simulink library "lib_EMachine"  (R2017b)
settings: Solver=VariableStepAuto  StartTime=0.0  StopTime=10.0  RelTol=1e-3
undefined symbols (not defined in the file): mot, t_amb, tloop
libraries: simulink x6, lib_Clutch x1
(part 1 of 2)
settings Model: Creator=Di Russo  LastModifiedBy=Vraj M
settings CodeAppCC: StateflowObjectComments=on

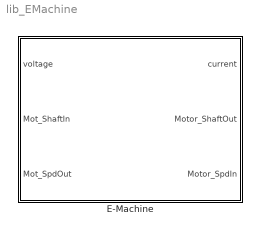
== system lib_EMachine ==
  E-Machine : Subsystem
      mask Display:
      | image('Images/motor.png')
      | color('red');
      | port_label('Input',1,'Volt');
      | port_label('Input',2,'ShaftIn');
      | port_label('Input',3,'SpdOut');
      | port_label('Output',1,'Crr');
      | port_label('Output',2,'ShaftOut');
      | port_label('Output',3,'SpdIn');

== system lib_EMachine/E-Machine ==
  voltage : Inport
  Mot_ShaftIn : Inport  Port=2
  Mot_SpdOut : Inport  Port=3
  Clutch Temporary 1 : Subsystem  Commented=on
  IMG Plant : Subsystem
      mask Display:
      | image('Images\Motor.png')
      | color('red');
      | port_label('Input',2,'Volt');
      | port_label('Input',3,'ShaftIn');
      | port_label('Input',4,'SpdOut');
      | port_label('Output',2,'Crr');
      | port_label('Output',3,'ShaftOut');
      | port_label('Output',4,'SpdIn');
  IMG Plant2 : Subsystem  Commented=on
      mask Display:
      | image('Images/motor.png')
      | color('red');
      | port_label('Input',2,'Volt');
      | port_label('Input',3,'SpdOut');
      | port_label('Input',1,'MCU_cmd');
      | port_label('Input',4,'ShaftIn');
      | port_label('Output',1,'Sensor_Out');
      | port_label('Output',2,'Crr');
      | port_label('Output',3,'MotTrqOut');
      | port_label('Output',4,'MotSpdIn');
  Soft MCU : Subsystem
      mask Display: image('SoftECU.jpg')
  current : Outport
  Motor_ShaftOut : Outport  Port=2
  Motor_SpdIn : Outport  Port=3
  tag scope: MCU_to_HCU=global
  wires:
  IMG Plant/4(SpdIn) -> Motor_SpdIn/1
  Mot_SpdOut/1 -> IMG Plant/4(SpdOut)
  Soft MCU/1(Out) -> [MCU_to_HCU]
  Soft MCU/2(Out1) -> IMG Plant/1("In1 ")  "MCU_to_Actuators"
  [HCU_to_HV_CAN] -> Soft MCU/1(In)
  IMG Plant/1(Out1) -> Soft MCU/2(In1)  "Sensors_to_MCU"
  Mot_ShaftIn/1 -> IMG Plant/3(MotShaftIn)
  IMG Plant/3(MotShaftOut) -> Motor_ShaftOut/1
  voltage/1 -> IMG Plant/2(voltage)
  IMG Plant/2(current) -> current/1

== system lib_EMachine/E-Machine/Clutch Temporary 1 ==
  In1 : Inport
  Constant : Constant  Value=0
  Memory : Memory
  Saturation : Saturate  UpperLimit=inf  LowerLimit=0
  Switch : Switch  Criteria=u2 > Threshold
  Out1 : Outport
  wires:
  Saturation/1 -> Memory/1
  Memory/1 -> Switch/1
  Constant/1 -> Switch/3
  In1/1 -> Saturation/1
  [cltch] -> Switch/2
  Switch/1 -> Out1/1

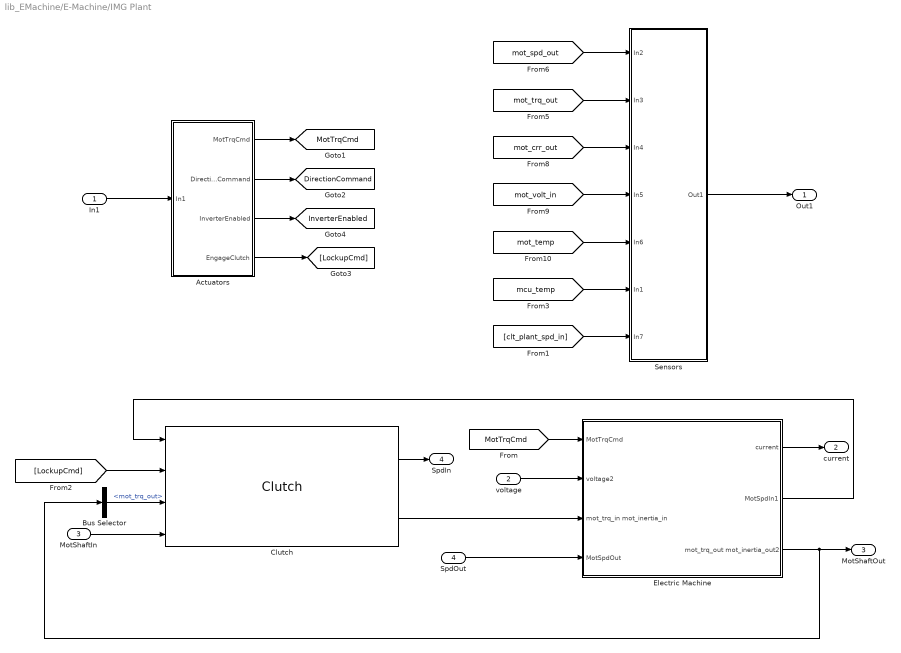
== system lib_EMachine/E-Machine/IMG Plant ==
  "In1 " : Inport
  voltage : Inport  Port=2
  MotShaftIn : Inport  Port=3
  SpdOut : Inport  Port=4
  " Actuators" : Subsystem
  Bus Selector : BusSelector  OutputSignals=mot_trq_out
  Clutch : lib_Clutch/Clutch  SystemSampleTime=-1
  Electric Machine : Subsystem
      mask Display:
      | image('Images\Motor.png')
      | color('red');
      | port_label('Input',1,'MotTrqCmd');
      | port_label('Input',2,'Volt');
      | port_label('Input',3,'ShaftIn');
      | port_label('Input',4,'SpdOut');
      | port_label('Output',1,'Crr')
      | port_label('Output',2,'SpdIn')
  Sensors : Subsystem
  Out1 : Outport
  current : Outport  Port=2
  MotShaftOut : Outport  Port=3
  SpdIn : Outport  Port=4
  tag scope: DirectionCommand=global, InverterEnabled=global, MotTrqCmd=global
  wires:
  Bus Selector/1 -> Clutch/3  "<mot_trq_out>"
  [mot_spd_out] -> Sensors/1(In2)
  [clt_plant_spd_in] -> Sensors/7(In7)
  Clutch/2 -> Electric Machine/3(mot_trq_in mot_inertia_in)
  SpdOut/1 -> Electric Machine/4(MotSpdOut)
  [mcu_temp] -> Sensors/6(In1)
  " Actuators"/3(InverterEnabled) -> [InverterEnabled]
  " Actuators"/2(DirectionCommand) -> [DirectionCommand]
  [LockupCmd] -> Clutch/2
  [mot_temp] -> Sensors/5(In6)
  [mot_crr_out] -> Sensors/3(In4)
  "In1 "/1 -> " Actuators"/1(In1)
  [mot_volt_in] -> Sensors/4(In5)
  " Actuators"/1(MotTrqCmd) -> [MotTrqCmd]
  Sensors/1(Out1) -> Out1/1
  [mot_trq_out] -> Sensors/2(In3)
  Clutch/1 -> SpdIn/1
  Electric Machine/3(mot_trq_out mot_inertia_out2) -> MotShaftOut/1, Bus Selector/1
  MotShaftIn/1 -> Clutch/4
  Electric Machine/2(MotSpdIn1) -> Clutch/1
  Electric Machine/1(current) -> current/1
  [MotTrqCmd] -> Electric Machine/1(MotTrqCmd)
  " Actuators"/4(EngageClutch) -> [LockupCmd]
  voltage/1 -> Electric Machine/2(voltage2)

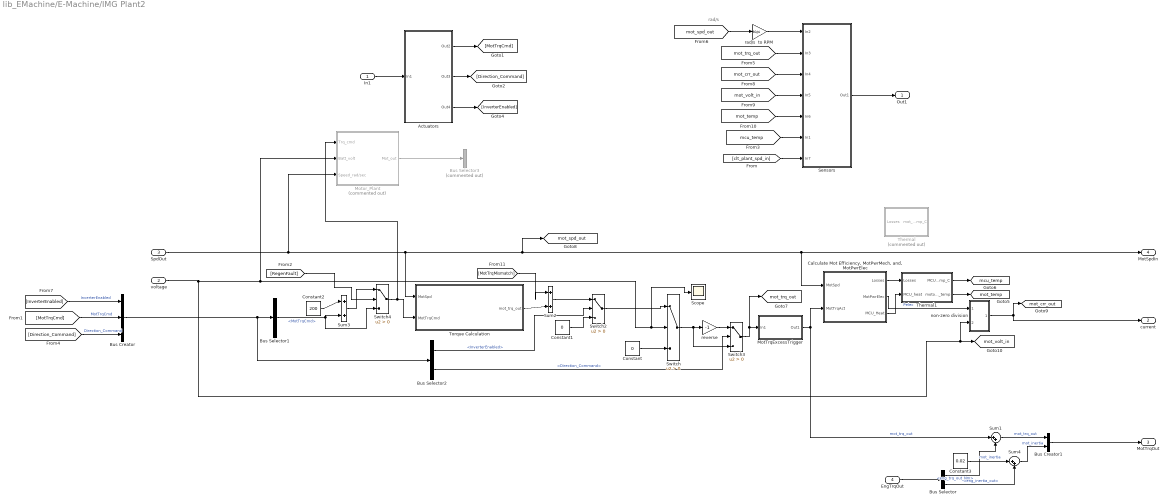
== system lib_EMachine/E-Machine/IMG Plant2 ==
  note: rad/s
  "In1 " : Inport
  voltage : Inport  Port=2
  SpdOut : Inport  Port=3
  EngTrqOut : Inport  Port=4
  " Actuators" : Subsystem
  Bus Creator : BusCreator  Inputs=3
  Bus Creator1 : BusCreator  Inputs=2
  Bus Selector : BusSelector  OutputSignals=eng_trq_out_Nm,eng_inertia_out
  Bus Selector1 : BusSelector  OutputSignals=MotTrqCmd
  Bus Selector2 : BusSelector  OutputSignals=InverterEnabled,Direction_Command
  Bus Selector3 : BusSelector  Commented=on  OutputSignals=Mot_current_A
  "Calculate Mot Efficiency, MotPwrMech, and, MotPwrElec" : Subsystem
  Constant : Constant  Value=0
  Constant1 : Constant  Value=0
  Constant2 : Constant  Value=200
  Constant3 : Constant  Value=0.02
  MotTrqExcessTrigger : Subsystem
  Motor_Plant : Subsystem  Commented=on
  Scope : Scope
  Sensors : Subsystem
  Sum{1..4} (4 alike) : Sum  Inputs=|++
  Switch{,2..4} (4 alike) : Switch  Criteria=u2 > Threshold
  Thermal : Subsystem  Commented=on
  Thermal1 : Subsystem
  Torque Calculation : Subsystem
  non-zero division : Subsystem
      mask Display: disp('divider \n I1/I2')
  rad/s  to RPM : Gain  Gain=30/pi
  reverse : Gain  Gain=-1
  Out1 : Outport
  current : Outport  Port=2
  MotTrqOut : Outport  Port=3
  MotSpdIn : Outport  Port=4
  tag scope: mcu_temp=global, mot_crr_out=global, mot_spd_out=global, mot_temp=global, mot_trq_out=global, mot_volt_in=global
  wires:
  [mot_temp] -> Sensors/5(In6)
  [mot_crr_out] -> Sensors/3(In4)
  "In1 "/1 -> " Actuators"/1(In1)
  [mot_volt_in] -> Sensors/4(In5)
  " Actuators"/1(Out2) -> [MotTrqCmd]
  Sensors/1(Out1) -> Out1/1
  [mot_trq_out] -> Sensors/2(In3)
  SpdOut/1 -> Motor_Plant/3(Speed_rad/sec), Torque Calculation/1(MotSpd), [mot_spd_out], MotSpdIn/1, "Calculate Mot Efficiency, MotPwrMech, and, MotPwrElec"/1(MotSpd)
  non-zero division/1(Out1) -> current/1, [mot_crr_out]
  [mcu_temp] -> Sensors/6(In1)
  [clt_plant_spd_in] -> Sensors/7(In7)
  " Actuators"/2(Out3) -> [Direction_Command]
  " Actuators"/3(Out4) -> [InverterEnabled]
  [Direction_Command] -> Bus Creator/3  "Direction_Command"
  [InverterEnabled] -> Bus Creator/1  "InverterEnabled"
  [MotTrqCmd] -> Bus Creator/2  "MotTrqCmd"
  [mot_spd_out] -> rad/s  to RPM/1
  rad/s  to RPM/1 -> Sensors/1(In2)
  Thermal1/1(MCU_temp_C) -> [mcu_temp]
  Constant2/1 -> Sum3/1
  Switch4/1 -> Motor_Plant/1(Trq_cmd), Torque Calculation/2(MotTrqCmd)
  Sum3/1 -> Switch4/1
  [RegenFault] -> Switch4/2
  Switch3/1 -> [mot_trq_out], MotTrqExcessTrigger/1(In1)
  reverse/1 -> Switch3/1
  Bus Selector2/2 -> Switch3/2  "<Direction_Command>"
  Switch2/1 -> Switch/1
  Constant1/1 -> Switch2/3
  Bus Selector2/1 -> Switch2/2  "<InverterEnabled>"
  Bus Selector1/1 -> Switch4/3, Sum3/2  "<MotTrqCmd>"
  Bus Creator/1 -> Bus Selector2/1, Bus Selector1/1
  Sum2/1 -> Switch2/1
  Torque Calculation/1(mot_trq_out) -> Sum2/2
  [MotTrqMismatch] -> Sum2/1
  Switch/1 -> Switch3/3, reverse/1
  Thermal1/2(motor_temp) -> [mot_temp]
  "Calculate Mot Efficiency, MotPwrMech, and, MotPwrElec"/3(MCU_Heat) -> Thermal1/2(MCU_heat)
  Constant/1 -> Switch/3
  "Calculate Mot Efficiency, MotPwrMech, and, MotPwrElec"/1(Losses) -> Thermal1/1(Losses)
  MotTrqExcessTrigger/1(Out1) -> Sum1/1, "Calculate Mot Efficiency, MotPwrMech, and, MotPwrElec"/2(MotTrqAct)  "mot_trq_out"
  "Calculate Mot Efficiency, MotPwrMech, and, MotPwrElec"/2(MotPwrElec) -> non-zero division/1(In1)  "Pelec"
  voltage/1 -> non-zero division/2(In2), [mot_volt_in], Motor_Plant/2(Batt_volt), Scope/1, Switch/2
  Bus Creator1/1 -> MotTrqOut/1
  Sum4/1 -> Bus Creator1/2  "mot_inertia"
  EngTrqOut/1 -> Bus Selector/1
  Sum1/1 -> Bus Creator1/1  "mot_trq_out"
  Bus Selector/2 -> Sum4/2  "<eng_inertia_out>"
  Constant3/1 -> Sum4/1  "mot_inertia"
  Bus Selector/1 -> Sum1/2  "<eng_trq_out_Nm>"
  Motor_Plant/1(Mot_out) -> Bus Selector3/1

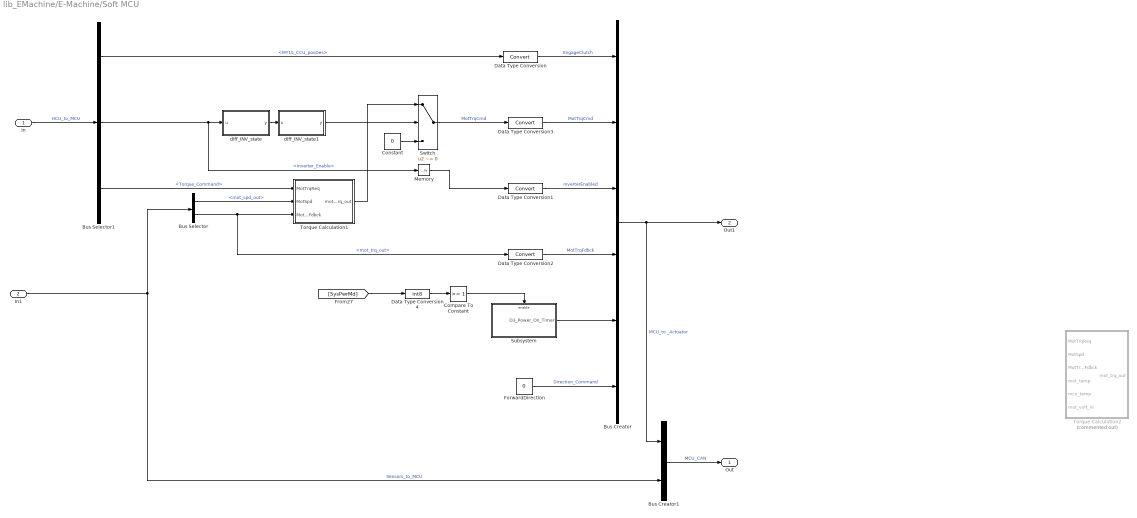
== system lib_EMachine/E-Machine/Soft MCU ==
  In : Inport
  In1 : Inport  Port=2
  Bus Creator : BusCreator  Inputs=6
  Bus Creator1 : BusCreator  Inputs=2
  Bus Selector : BusSelector  OutputSignals=mot_spd_out,mot_trq_out
  Bus Selector1 : BusSelector  OutputSignals=MSG_HYB_115.MY15_CCU_posDes,M192_Command_Message.Inverter_Enable,M192_Command_Message.Torque_Command
  Compare To Constant : simulink/Logic and Bit Operations/Compare To Constant  relop=>=  const=1  OutDataTypeStr=boolean
  Constant : Constant  Value=0
  Data Type Conversion{,1..3} (4 alike) : DataTypeConversion
  Data Type Conversion4 : DataTypeConversion  OutDataTypeStr=int8
  ForwardDirection : Constant  Value=0
  Memory : Memory
  Subsystem : Subsystem
  Switch : Switch  Criteria=u2 ~= 0  Threshold=1
  Torque Calculation1 : Subsystem
  Torque Calculation2 : Subsystem  Commented=on
  diff_INV_state : MATLAB Function  TreatAsAtomicUnit=on
  diff_INV_state1 : MATLAB Function  TreatAsAtomicUnit=on
  Out : Outport
  Out1 : Outport  Port=2
  wires:
  Compare To Constant/1 -> Subsystem/Enable
  Subsystem/1(D3_Power_On_Timer) -> Bus Creator/5
  [SysPwrMd] -> Data Type Conversion4/1
  Data Type Conversion4/1 -> Compare To Constant/1
  Torque Calculation1/1(mot_trq_out) -> Switch/1
  diff_INV_state1/1(y) -> Switch/2
  Bus Selector1/2 -> diff_INV_state/1(u), Memory/1  "<Inverter_Enable>"
  diff_INV_state/1(y) -> diff_INV_state1/1(u)
  ForwardDirection/1 -> Bus Creator/6  "Direction_Command"
  Data Type Conversion3/1 -> Bus Creator/2  "MotTrqCmd"
  Switch/1 -> Data Type Conversion3/1  "MotTrqCmd"
  Memory/1 -> Data Type Conversion1/1
  Data Type Conversion2/1 -> Bus Creator/4  "MotTrqFdbck"
  Bus Selector/2 -> Data Type Conversion2/1, Torque Calculation1/3(MotTrqFdbck)  "<mot_trq_out>"
  Data Type Conversion1/1 -> Bus Creator/3  "InverterEnabled"
  Bus Selector/1 -> Torque Calculation1/2(MotSpd)  "<mot_spd_out>"
  Data Type Conversion/1 -> Bus Creator/1  "EngageClutch"
  Bus Selector1/1 -> Data Type Conversion/1  "<MY15_CCU_posDes>"
  Constant/1 -> Switch/3
  Bus Creator/1 -> Out1/1, Bus Creator1/1  "MCU_to _Actuator"
  Bus Selector1/3 -> Torque Calculation1/1(MotTrqReq)  "<Torque_Command>"
  In/1 -> Bus Selector1/1  "HCU_to_MCU"
  Bus Creator1/1 -> Out/1  "MCU_CAN"
  In1/1 -> Bus Creator1/2, Bus Selector/1  "Sensors_to_MCU"

== system lib_EMachine/E-Machine/IMG Plant/ Actuators ==
  In1 : Inport
  Bus Selector : BusSelector  OutputSignals=MotTrqCmd,Direction_Command,InverterEnabled,EngageClutch
  MotTrqCmd : Outport
  DirectionCommand : Outport  Port=2
  InverterEnabled : Outport  Port=3
  EngageClutch : Outport  Port=4
  wires:
  Bus Selector/3 -> InverterEnabled/1  "<InverterEnabled>"
  Bus Selector/2 -> DirectionCommand/1  "<Direction_Command>"
  Bus Selector/1 -> MotTrqCmd/1  "<MotTrqCmd>"
  In1/1 -> Bus Selector/1
  Bus Selector/4 -> EngageClutch/1  "<EngageClutch>"

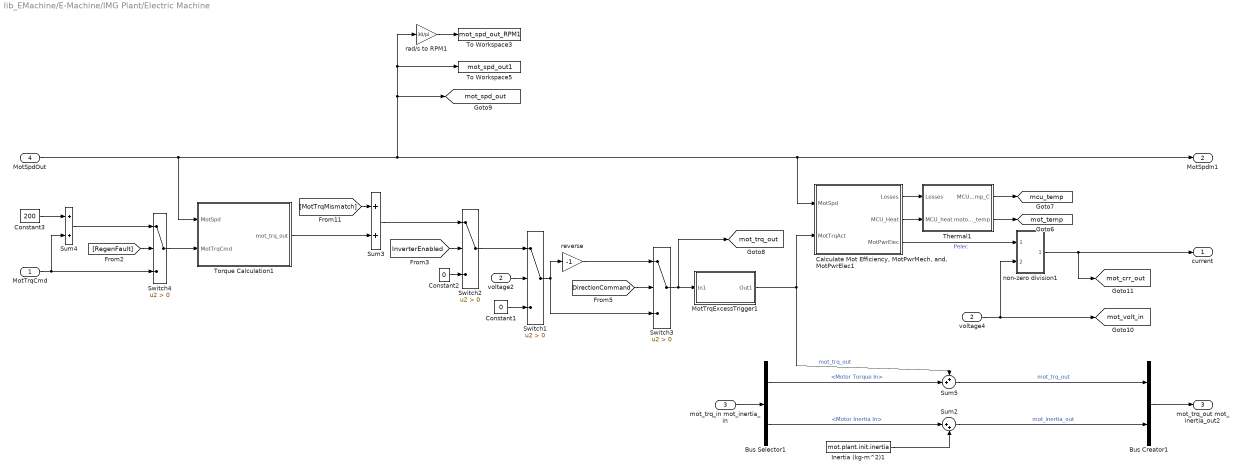
== system lib_EMachine/E-Machine/IMG Plant/Electric Machine ==
  MotTrqCmd : Inport
  voltage2 : Inport  Port=2
  mot_trq_in mot_inertia_in : Inport  Port=3
  MotSpdOut : Inport  Port=4
  Bus Creator1 : BusCreator  Inputs=2
  Bus Selector1 : BusSelector  OutputSignals=Motor Torque In,Motor Inertia In
  "Calculate Mot Efficiency, MotPwrMech, and, MotPwrElec1" : Subsystem
  Constant1 : Constant  Value=0
  Constant2 : Constant  Value=0
  Constant3 : Constant  Value=200
  Inertia (kg-m^2)1 : Constant  Value=mot.plant.init.inertia
  MotTrqExcessTrigger1 : Subsystem
  Sum2 : Sum  Inputs=|++
  Sum3 : Sum
  Sum4 : Sum
  Sum5 : Sum  Inputs=++|
  Switch{1..4} (4 alike) : Switch  Criteria=u2 > Threshold
  Thermal1 : Subsystem
  To Workspace3 : ToWorkspace  VariableName=mot_spd_out_RPM1  SampleTime=-1
      settings: Decimation=WORKSPACE_DECIMATION
  To Workspace5 : ToWorkspace  VariableName=mot_spd_out1  SampleTime=-1
      settings: Decimation=WORKSPACE_DECIMATION
  Torque Calculation1 : Subsystem
  non-zero division1 : Subsystem
      mask Display: disp('divider \n I1/I2')
  rad/s to RPM1 : Gain  Gain=30/pi
  reverse : Gain  Gain=-1
  voltage4 : InportShadow  Port=2
  current : Outport
  MotSpdIn1 : Outport  Port=2
  mot_trq_out mot_inertia_out2 : Outport  Port=3
  tag scope: mcu_temp=global, mot_crr_out=global, mot_spd_out=global, mot_temp=global, mot_trq_out=global, mot_volt_in=global
  wires:
  MotSpdOut/1 -> Torque Calculation1/1(MotSpd), [mot_spd_out], rad/s to RPM1/1, To Workspace5/1, MotSpdIn1/1, "Calculate Mot Efficiency, MotPwrMech, and, MotPwrElec1"/1(MotSpd)
  rad/s to RPM1/1 -> To Workspace3/1
  Bus Selector1/1 -> Sum5/2  "<Motor Torque In>"
  Bus Selector1/2 -> Sum2/1  "<Motor Inertia In>"
  mot_trq_in mot_inertia_in/1 -> Bus Selector1/1
  Bus Creator1/1 -> mot_trq_out mot_inertia_out2/1
  Sum2/1 -> Bus Creator1/2  "mot_inertia_out"
  Inertia (kg-m^2)1/1 -> Sum2/2
  Sum5/1 -> Bus Creator1/1  "mot_trq_out"
  [DirectionCommand] -> Switch3/2
  [InverterEnabled] -> Switch2/2
  [MotTrqMismatch] -> Sum3/1
  voltage4/1 -> [mot_volt_in], non-zero division1/2(In2)
  voltage2/1 -> Switch1/2
  Constant1/1 -> Switch1/3
  Switch1/1 -> Switch3/3, reverse/1
  Constant2/1 -> Switch2/3
  MotTrqCmd/1 -> Switch4/3, Sum4/2
  Sum3/1 -> Switch2/1
  MotTrqExcessTrigger1/1(Out1) -> "Calculate Mot Efficiency, MotPwrMech, and, MotPwrElec1"/2(MotTrqAct), Sum5/1  "mot_trq_out"
  non-zero division1/1(Out1) -> current/1, [mot_crr_out]
  reverse/1 -> Switch3/1
  "Calculate Mot Efficiency, MotPwrMech, and, MotPwrElec1"/3(MotPwrElec) -> non-zero division1/1(In1)  "Pelec"
  Switch4/1 -> Torque Calculation1/2(MotTrqCmd)
  "Calculate Mot Efficiency, MotPwrMech, and, MotPwrElec1"/2(MCU_Heat) -> Thermal1/2(MCU_heat)
  Switch3/1 -> [mot_trq_out], MotTrqExcessTrigger1/1(In1)
  Sum4/1 -> Switch4/1
  "Calculate Mot Efficiency, MotPwrMech, and, MotPwrElec1"/1(Losses) -> Thermal1/1(Losses)
  [RegenFault] -> Switch4/2
  Switch2/1 -> Switch1/1
  Torque Calculation1/1(mot_trq_out) -> Sum3/2
  Constant3/1 -> Sum4/1
  Thermal1/2(motor_temp) -> [mot_temp]
  Thermal1/1(MCU_temp_C) -> [mcu_temp]

== system lib_EMachine/E-Machine/IMG Plant/Sensors ==
  In2 : Inport
  In3 : Inport  Port=2
  In4 : Inport  Port=3
  In5 : Inport  Port=4
  In6 : Inport  Port=5
  In1 : Inport  Port=6
  In7 : Inport  Port=7
  Bus Creator : BusCreator  Inputs=7
  Out1 : Outport
  wires:
  In7/1 -> Bus Creator/7  "clt_plant_spd_in"
  In1/1 -> Bus Creator/6  "mcu_temp"
  In6/1 -> Bus Creator/5  "mot_temp"
  In3/1 -> Bus Creator/2  "mot_trq_out"
  In5/1 -> Bus Creator/4  "mot_volt_in"
  In4/1 -> Bus Creator/3  "mot_crr_out"
  In2/1 -> Bus Creator/1  "mot_spd_out"
  Bus Creator/1 -> Out1/1

== system lib_EMachine/E-Machine/IMG Plant2/ Actuators ==
  In1 : Inport
  Bus Selector : BusSelector  OutputSignals=MotTrqCmd,Direction_Command,InverterEnabled
  Out2 : Outport
  Out3 : Outport  Port=2
  Out4 : Outport  Port=3
  wires:
  Bus Selector/1 -> Out2/1  "<MotTrqCmd>"
  In1/1 -> Bus Selector/1
  Bus Selector/2 -> Out3/1  "<Direction_Command>"
  Bus Selector/3 -> Out4/1  "<InverterEnabled>"

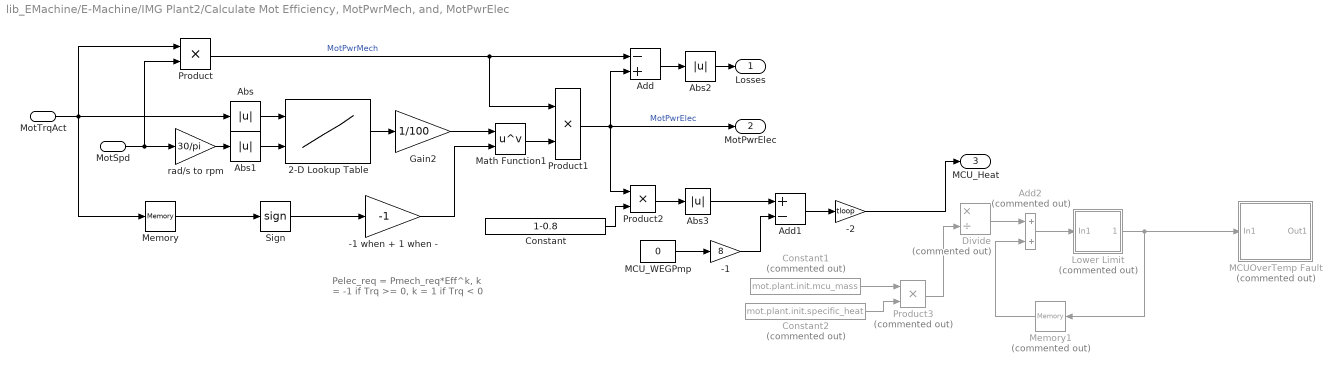
== system lib_EMachine/E-Machine/IMG Plant2/Calculate Mot Efficiency, MotPwrMech, and, MotPwrElec ==
  note: Pelec_req = Pmech_req*Eff^k,
      | k = -1 if Trq >= 0,
      | k = 1 if Trq < 0
  MotSpd : Inport
  MotTrqAct : Inport  Port=2
  -1 : Gain  Gain=8
  "-1 when + 1 when - " : Gain  Gain=-1
  -2 : Gain  Gain=tloop
  2-D Lookup Table : Lookup_n-D  BreakpointsForDimension1=mot.plant.init.eff_trq.idx2_trq  BreakpointsForDimension2=mot.plant.init.eff_trq.idx1_spd  Table=mot.plant.init.eff_trq.map  InternalRulePriority=Speed  RndMeth=Simplest  InputSameDT=on
  Abs{,1..3} (4 alike) : Abs
  Add : Sum  Inputs=-+
  Add1 : Sum  Inputs=+-
  Add2 : Sum  Commented=on
  Constant : Constant  Value=1-0.8
  Constant1 : Constant  Commented=on  Value=mot.plant.init.mcu_mass
  Constant2 : Constant  Commented=on  Value=mot.plant.init.specific_heat
  Divide : Product  Commented=on  Inputs=*/
  Gain2 : Gain  Gain=1/100
  Lower Limit : Subsystem  Commented=on  mask{Lolimit=t_amb+20}
      mask prompts: Lolimit "Lower Limit"
  MCUOverTemp Fault : Subsystem  Commented=on
  MCU_WEGPmp : Constant  Value=0
  Math Function1 : Math  Operator=pow  SaturateOnIntegerOverflow=on
  Memory : Memory
  Memory1 : Memory  Commented=on
  Product : Product
  Product1 : Product
  Product2 : Product
  Product3 : Product  Commented=on
  Sign : Signum
  rad/s to rpm : Gain  Gain=30/pi
  Losses : Outport
  MotPwrElec : Outport  Port=2
  MCU_Heat : Outport  Port=3
  wires:
  rad/s to rpm/1 -> Abs1/1
  Abs1/1 -> 2-D Lookup Table/2
  Sign/1 -> "-1 when + 1 when - "/1
  Abs/1 -> 2-D Lookup Table/1
  Gain2/1 -> Math Function1/1
  2-D Lookup Table/1 -> Gain2/1
  Product1/1 -> Product2/1, Add/2, MotPwrElec/1  "MotPwrElec"
  Product/1 -> Add/1, Product1/1  "MotPwrMech"
  MotTrqAct/1 -> Memory/1, Product/1, Abs/1
  MotSpd/1 -> Product/2, rad/s to rpm/1
  "-1 when + 1 when - "/1 -> Math Function1/2
  Abs2/1 -> Losses/1
  Add/1 -> Abs2/1
  Math Function1/1 -> Product1/2
  Memory/1 -> Sign/1
  Constant/1 -> Product2/2
  Product2/1 -> Abs3/1
  Abs3/1 -> Add1/1
  MCU_WEGPmp/1 -> -1/1
  Add1/1 -> -2/1
  -1/1 -> Add1/2
  -2/1 -> MCU_Heat/1
  Constant1/1 -> Product3/1
  Constant2/1 -> Product3/2
  Product3/1 -> Divide/2
  Divide/1 -> Add2/1
  Memory1/1 -> Add2/2
  Add2/1 -> Lower Limit/1(In1)
  Lower Limit/1(Out1) -> MCUOverTemp Fault/1(In1), Memory1/1

== system lib_EMachine/E-Machine/IMG Plant2/MotTrqExcessTrigger ==
  In1 : Inport
  Bias : Bias  Bias=55
  Bias1 : Bias  Bias=25
  Constant : Constant  Value=0
  Multiport Switch : MultiPortSwitch  DataPortOrder=Zero-based contiguous
  Out1 : Outport
  tag scope: MotTrqExcessTrig=global
  wires:
  Multiport Switch/1 -> Out1/1
  Bias/1 -> Multiport Switch/4
  In1/1 -> Multiport Switch/2, Bias/1, Bias1/1
  Bias1/1 -> Multiport Switch/3
  Constant/1 -> [MotTrqExcessTrig], Multiport Switch/1

== system lib_EMachine/E-Machine/IMG Plant2/Motor_Plant ==
  Trq_cmd : Inport
  Batt_volt : Inport  Port=2
  Speed_rad/sec : Inport  Port=3
  Add : Sum
  Bus Creator : BusCreator  Inputs=5
  Efficiency Calcs : Subsystem
  Memory : Memory
  Random Number : RandomNumber  Mean=0.1  Variance=0.1  SampleTime=0.01
  rad/sec to rpm : Gain  Gain=60/(2*3.14)
  Mot_out : Outport
  wires:
  Add/1 -> Memory/1
  Speed_rad/sec/1 -> rad/sec to rpm/1
  rad/sec to rpm/1 -> Bus Creator/2, Efficiency Calcs/1(Speed_rpm)  "Mot_spd_rpm"
  Random Number/1 -> Add/2
  Memory/1 -> Bus Creator/1, Efficiency Calcs/2(Torq_cmd_Nm)  "Mot_Trq_Nm"
  Bus Creator/1 -> Mot_out/1
  Trq_cmd/1 -> Add/1
  Batt_volt/1 -> Efficiency Calcs/3(Batt_volt)
  Efficiency Calcs/1(Mot_current) -> Bus Creator/3
  Efficiency Calcs/2(Mech_power_W) -> Bus Creator/4
  Efficiency Calcs/3(Elec_power_W) -> Bus Creator/5

== system lib_EMachine/E-Machine/IMG Plant2/Sensors ==
  In2 : Inport
  In3 : Inport  Port=2
  In4 : Inport  Port=3
  In5 : Inport  Port=4
  In6 : Inport  Port=5
  In1 : Inport  Port=6
  In7 : Inport  Port=7
  Bus Creator : BusCreator  Inputs=7
  Out1 : Outport
  wires:
  In6/1 -> Bus Creator/5  "mot_temp"
  In3/1 -> Bus Creator/2  "mot_trq_out"
  In5/1 -> Bus Creator/4  "mot_volt_in"
  In4/1 -> Bus Creator/3  "mot_crr_out"
  In2/1 -> Bus Creator/1  "mot_spd_out"
  Bus Creator/1 -> Out1/1
  In1/1 -> Bus Creator/6  "mcu_temp"
  In7/1 -> Bus Creator/7  "clt_plant_spd_in"

== system lib_EMachine/E-Machine/IMG Plant2/Thermal ==
  Losses : Inport
  Motor Thermal : Subsystem
  mot_temp_C : Outport
  wires:
  Losses/1 -> Motor Thermal/1(In1)  "[W]"
  Motor Thermal/1(Out1) -> mot_temp_C/1

== system lib_EMachine/E-Machine/IMG Plant2/Thermal1 ==
  Losses : Inport
  MCU_heat : Inport  Port=2
  MotInv_loop : Subsystem
  Motor Thermal : Subsystem  Commented=on
  MCU_temp_C : Outport
  motor_temp : Outport  Port=2
  wires:
  MCU_heat/1 -> MotInv_loop/2(In2)
  Losses/1 -> MotInv_loop/1(In1)  "[W]"
  MotInv_loop/1(Out1) -> MCU_temp_C/1
  MotInv_loop/2(Out2) -> motor_temp/1

== system lib_EMachine/E-Machine/IMG Plant2/Torque Calculation ==
  MotSpd : Inport
  MotTrqCmd : Inport  Port=2
  Abs : Abs
  Abs1 : Abs
  MinMax : MinMax  Inputs=2
  Product : Product
  Sign : Signum
  electric machine filter : Subsystem
  "max torque " : Subsystem
  mot_trq_out : Outport
  wires:
  "max torque "/1(max torque) -> Abs1/1
  MotSpd/1 -> "max torque "/2(speed)
  Sign/1 -> Product/1
  MinMax/1 -> Product/2
  Abs/1 -> MinMax/1
  Abs1/1 -> MinMax/2
  electric machine filter/1(filtered) -> mot_trq_out/1
  MotTrqCmd/1 -> "max torque "/1(cmd), Sign/1, Abs/1
  Product/1 -> electric machine filter/1(trq)

== system lib_EMachine/E-Machine/IMG Plant2/non-zero division ==
  note: original idea from Phil Sharer - ANL
      | original formula: u[1]\(u[2]+eps)*(u[2]!=0)
      | changes done by Gerald ZINI (dgey) - ANL (05\02\2001)
  note: (u[2]==0) is true then returns 1, thus (u[2]+(u[2]==0)) is equal to 0+1=1
  note: if u[2] == 0, then output == 0:
  note: (u[2]!=0) is false then returns 0
  note: and finally, the expression is: (u[1] \ 1) * 0 = 0
  note: (u[2]==0) is false then returns 0, thus (u[2]+(u[2]==0)) is equal to u[2]+0=u[2]
  note: if u[2] != 0, then output == u[1]\u[2]:
  note: (u[2]!=0) is true then returns 1
  note: and finally, the expression is: (u[1] \ u[2]) * 1 = u[1] \ u[2]
  In1 : Inport
  In2 : Inport  Port=2
  Fcn : Fcn  Expr=u[1]/(u[2]+(u[2]==0))*(u[2]!=0)
  Mux : Mux  Inputs=2
  Out1 : Outport
  wires:
  Mux/1 -> Fcn/1
  In1/1 -> Mux/1
  Fcn/1 -> Out1/1
  In2/1 -> Mux/2

== system lib_EMachine/E-Machine/Soft MCU/Subsystem ==
  Enable : EnablePort
  MCU_RollingAliveCnt : Subsystem
  D3_Power_On_Timer : Outport
  wires:
  MCU_RollingAliveCnt/1(Out1) -> D3_Power_On_Timer/1  "D3_Power_On_Timer"

== system lib_EMachine/E-Machine/Soft MCU/Torque Calculation1 ==
  MotTrqReq : Inport
  MotSpd : Inport  Port=2
  MotTrqFdbck : Inport  Port=3
  Abs : Abs
  Abs1 : Abs
  MinMax : MinMax  Inputs=2
  Product : Product
  Sign : Signum
  "max torque " : Subsystem
  mot_trq_out : Outport
  wires:
  MotTrqFdbck/1 -> "max torque "/3(torque)
  Abs1/1 -> MinMax/2
  Abs/1 -> MinMax/1
  MinMax/1 -> Product/2
  Sign/1 -> Product/1
  MotTrqReq/1 -> Abs/1, Sign/1, "max torque "/1(Req)
  MotSpd/1 -> "max torque "/2(speed)
  "max torque "/1(max torque) -> Abs1/1
  Product/1 -> mot_trq_out/1

== system lib_EMachine/E-Machine/Soft MCU/Torque Calculation2 ==
  MotTrqReq : Inport
  MotSpd : Inport  Port=2
  MotTrqFdbck : Inport  Port=3
  mot_temp : Inport  Port=4
  mcu_temp : Inport  Port=5
  mot_volt_in : Inport  Port=6
  1-D Lookup Table : Lookup_n-D  NumberOfTableDimensions=1  BreakpointsForDimension1=[0,12600,12700,12800,12900,13000]  Table=[1,1,0.75,0.5,0.25,0]  InternalRulePriority=Speed  RndMeth=Simplest  InputSameDT=on
  1-D Lookup Table1 : Lookup_n-D  NumberOfTableDimensions=1  BreakpointsForDimension1=[0,410,415,420,425,430]  Table=[1,1,0.75,0.5,0.25,0]  InternalRulePriority=Speed  RndMeth=Simplest  InputSameDT=on
  1-D Lookup Table2 : Lookup_n-D  Commented=on  NumberOfTableDimensions=1  BreakpointsForDimension1=[0,90,100]  Table=[1,1,0]  InternalRulePriority=Speed  RndMeth=Simplest  InputSameDT=on
  1-D Lookup Table3 : Lookup_n-D  NumberOfTableDimensions=1  BreakpointsForDimension1=[0,150,170]  Table=[1,1,0]  InternalRulePriority=Speed  RndMeth=Simplest  InputSameDT=on
  Abs : Abs
  Abs1 : Abs
  Constant : Constant
  MinMax : MinMax  Inputs=2
  Product : Product
  Product1 : Product  Inputs=5
  Sign : Signum
  Terminator1 : Terminator
  "max torque " : Subsystem
  rad/s to RPM1 : Gain  Gain=30/pi
  mot_trq_out : Outport
  wires:
  1-D Lookup Table3/1 -> Product1/1
  Constant/1 -> Product1/2
  mcu_temp/1 -> Terminator1/1
  mot_temp/1 -> 1-D Lookup Table3/1
  1-D Lookup Table1/1 -> Product1/3
  mot_volt_in/1 -> 1-D Lookup Table1/1
  1-D Lookup Table/1 -> Product1/4
  Product1/1 -> mot_trq_out/1
  rad/s to RPM1/1 -> 1-D Lookup Table/1
  MotTrqFdbck/1 -> "max torque "/3(torque)
  Abs1/1 -> MinMax/2
  Abs/1 -> MinMax/1
  MinMax/1 -> Product/2
  Sign/1 -> Product/1
  MotTrqReq/1 -> Abs/1, Sign/1, "max torque "/1(Req)
  MotSpd/1 -> "max torque "/2(speed), rad/s to RPM1/1
  "max torque "/1(max torque) -> Abs1/1
  Product/1 -> Product1/5

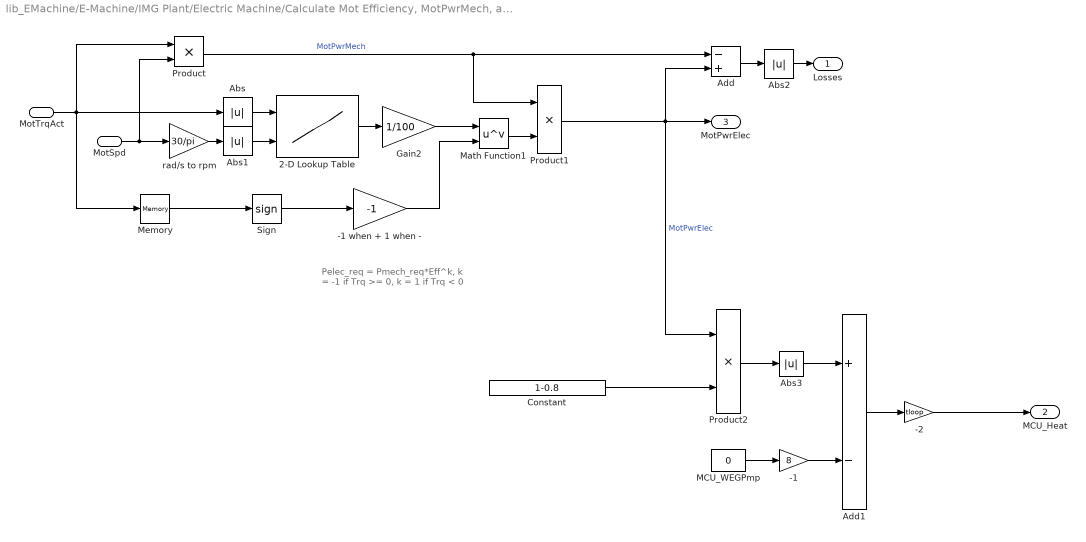
== system lib_EMachine/E-Machine/IMG Plant/Electric Machine/Calculate Mot Efficiency, MotPwrMech, and, MotPwrElec1 ==
  note: Pelec_req = Pmech_req*Eff^k,
      | k = -1 if Trq >= 0,
      | k = 1 if Trq < 0
  MotSpd : Inport
  MotTrqAct : Inport  Port=2
  -1 : Gain  Gain=8
  "-1 when + 1 when - " : Gain  Gain=-1
  -2 : Gain  Gain=tloop
  2-D Lookup Table : Lookup_n-D  BreakpointsForDimension1=mot.plant.init.eff_trq.idx2_trq  BreakpointsForDimension2=mot.plant.init.eff_trq.idx1_spd  Table=mot.plant.init.eff_trq.map  InternalRulePriority=Speed  RndMeth=Simplest  InputSameDT=on
  Abs{,1..3} (4 alike) : Abs
  Add : Sum  Inputs=-+
  Add1 : Sum  Inputs=+-
  Constant : Constant  Value=1-0.8
  Gain2 : Gain  Gain=1/100
  MCU_WEGPmp : Constant  Value=0
  Math Function1 : Math  Operator=pow  SaturateOnIntegerOverflow=on
  Memory : Memory
  Product : Product
  Product1 : Product
  Product2 : Product
  Sign : Signum
  rad/s to rpm : Gain  Gain=30/pi
  Losses : Outport
  MCU_Heat : Outport  Port=2
  MotPwrElec : Outport  Port=3
  wires:
  rad/s to rpm/1 -> Abs1/1
  Abs1/1 -> 2-D Lookup Table/2
  Sign/1 -> "-1 when + 1 when - "/1
  Abs/1 -> 2-D Lookup Table/1
  Gain2/1 -> Math Function1/1
  2-D Lookup Table/1 -> Gain2/1
  Product1/1 -> MotPwrElec/1, Product2/1, Add/2  "MotPwrElec"
  Product/1 -> Add/1, Product1/1  "MotPwrMech"
  MotTrqAct/1 -> Memory/1, Product/1, Abs/1
  MotSpd/1 -> Product/2, rad/s to rpm/1
  "-1 when + 1 when - "/1 -> Math Function1/2
  Abs2/1 -> Losses/1
  Add/1 -> Abs2/1
  Math Function1/1 -> Product1/2
  Memory/1 -> Sign/1
  Constant/1 -> Product2/2
  Product2/1 -> Abs3/1
  Abs3/1 -> Add1/1
  MCU_WEGPmp/1 -> -1/1
  Add1/1 -> -2/1
  -1/1 -> Add1/2
  -2/1 -> MCU_Heat/1

== system lib_EMachine/E-Machine/IMG Plant/Electric Machine/MotTrqExcessTrigger1 ==
  In1 : Inport
  Bias : Bias  Bias=55
  Bias1 : Bias  Bias=25
  Constant : Constant  Value=0
  Multiport Switch : MultiPortSwitch  DataPortOrder=Zero-based contiguous
  Terminator : Terminator
  Out1 : Outport
  tag scope: MotTrqExcessTrig=global
  wires:
  [MotTrqExcessTrig] -> Terminator/1
  Multiport Switch/1 -> Out1/1
  Bias/1 -> Multiport Switch/4
  In1/1 -> Multiport Switch/2, Bias/1, Bias1/1
  Bias1/1 -> Multiport Switch/3
  Constant/1 -> [MotTrqExcessTrig], Multiport Switch/1

== system lib_EMachine/E-Machine/IMG Plant/Electric Machine/Thermal1 ==
  Losses : Inport
  MCU_heat : Inport  Port=2
  MotInv_loop : Subsystem
  Motor Thermal : Subsystem  Commented=on
  MCU_temp_C : Outport
  motor_temp : Outport  Port=2
  wires:
  MCU_heat/1 -> MotInv_loop/2(In2)
  Losses/1 -> MotInv_loop/1(In1)  "[W]"
  MotInv_loop/1(Out1) -> MCU_temp_C/1
  MotInv_loop/2(Out2) -> motor_temp/1

== system lib_EMachine/E-Machine/IMG Plant/Electric Machine/Torque Calculation1 ==
  MotSpd : Inport
  MotTrqCmd : Inport  Port=2
  Abs : Abs
  Abs1 : Abs
  Memory : Memory
  MinMax : MinMax  Inputs=2
  Product : Product
  Sign : Signum
  electric machine filter : Subsystem
  "max torque " : Subsystem
  mot_trq_out : Outport
  wires:
  Memory/1 -> electric machine filter/1(trq)
  "max torque "/1(max torque) -> Abs1/1
  MotSpd/1 -> "max torque "/2(speed)
  Sign/1 -> Product/1
  MinMax/1 -> Product/2
  Abs/1 -> MinMax/1
  Abs1/1 -> MinMax/2
  electric machine filter/1(filtered) -> mot_trq_out/1
  MotTrqCmd/1 -> "max torque "/1(cmd), Sign/1, Abs/1
  Product/1 -> Memory/1

== system lib_EMachine/E-Machine/IMG Plant/Electric Machine/non-zero division1 ==
  note: original idea from Phil Sharer - ANL
      | original formula: u[1]\(u[2]+eps)*(u[2]!=0)
      | changes done by Gerald ZINI (dgey) - ANL (05\02\2001)
  note: (u[2]==0) is true then returns 1, thus (u[2]+(u[2]==0)) is equal to 0+1=1
  note: if u[2] == 0, then output == 0:
  note: (u[2]!=0) is false then returns 0
  note: and finally, the expression is: (u[1] \ 1) * 0 = 0
  note: (u[2]==0) is false then returns 0, thus (u[2]+(u[2]==0)) is equal to u[2]+0=u[2]
  note: if u[2] != 0, then output == u[1]\u[2]:
  note: (u[2]!=0) is true then returns 1
  note: and finally, the expression is: (u[1] \ u[2]) * 1 = u[1] \ u[2]
  In1 : Inport
  In2 : Inport  Port=2
  Fcn : Fcn  Expr=u[1]/(u[2]+(u[2]==0))*(u[2]!=0)
  Mux : Mux  Inputs=2
  Out1 : Outport
  wires:
  Mux/1 -> Fcn/1
  In1/1 -> Mux/1
  Fcn/1 -> Out1/1
  In2/1 -> Mux/2

== system lib_EMachine/E-Machine/IMG Plant2/Calculate Mot Efficiency, MotPwrMech, and, MotPwrElec/Lower Limit ==
  In1 : Inport
  Constant3 : Constant  Value=Lolimit
  MinMax : MinMax  Function=max  Inputs=2
  Out1 : Outport
  wires:
  In1/1 -> MinMax/1
  Constant3/1 -> MinMax/2
  MinMax/1 -> Out1/1

== system lib_EMachine/E-Machine/IMG Plant2/Calculate Mot Efficiency, MotPwrMech, and, MotPwrElec/MCUOverTemp Fault ==
  In1 : Inport
  Gain : Gain  Gain=3
  Switch : Switch  Threshold=1
  Out1 : Outport
  wires:
  In1/1 -> Switch/3, Gain/1
  [MCUOverTemp] -> Switch/2
  Gain/1 -> Switch/1
  Switch/1 -> Out1/1

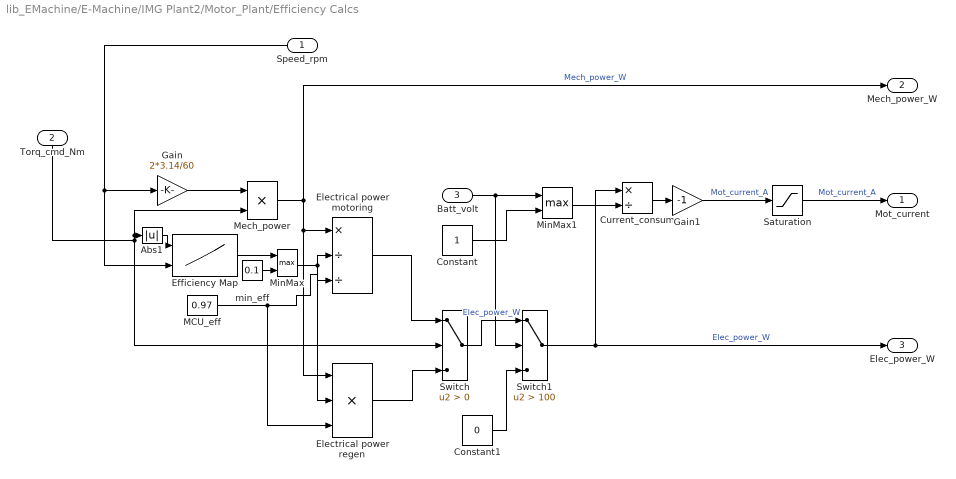
== system lib_EMachine/E-Machine/IMG Plant2/Motor_Plant/Efficiency Calcs ==
  Speed_rpm : Inport
  Torq_cmd_Nm : Inport  Port=2
  Batt_volt : Inport  Port=3
  Abs1 : Abs
  Constant : Constant
  Constant1 : Constant  Value=0
  Current_consum : Product  Inputs=*/
  Efficiency Map : Lookup_n-D  BreakpointsForDimension1=mot.map.trqindex  BreakpointsForDimension2=mot.map.spdindex  Table=mot.map.eff  InternalRulePriority=Speed  RndMeth=Simplest  InputSameDT=on
  Electrical power motoring : Product  Inputs=*//
  Electrical power regen : Product  Inputs=***
  Gain : Gain  Gain=2*3.14/60
  Gain1 : Gain  Gain=-1
  MCU_eff : Constant  Value=0.97
  Mech_power : Product  Inputs=**
  MinMax : MinMax  Function=max  Inputs=2
  MinMax1 : MinMax  Function=max  Inputs=2
  Saturation : Saturate  UpperLimit=400  LowerLimit=-400
  Switch : Switch  Criteria=u2 > Threshold
  Switch1 : Switch  Criteria=u2 > Threshold  Threshold=100
  min_eff : Constant  Value=0.1
  Mot_current : Outport
  Mech_power_W : Outport  Port=2
  Elec_power_W : Outport  Port=3
  wires:
  Speed_rpm/1 -> Efficiency Map/2, Gain/1
  Torq_cmd_Nm/1 -> Mech_power/2, Abs1/1, Switch/2
  Electrical power regen/1 -> Switch/3
  MinMax/1 -> Electrical power motoring/2, Electrical power regen/2
  Current_consum/1 -> Gain1/1
  Saturation/1 -> Mot_current/1  "Mot_current_A"
  Gain/1 -> Mech_power/1
  Batt_volt/1 -> Switch1/2, MinMax1/1
  Abs1/1 -> Efficiency Map/1
  Mech_power/1 -> Electrical power motoring/1, Electrical power regen/1, Mech_power_W/1  "Mech_power_W"
  MCU_eff/1 -> Electrical power regen/3, Electrical power motoring/3
  Electrical power motoring/1 -> Switch/1
  min_eff/1 -> MinMax/2
  Switch1/1 -> Elec_power_W/1, Current_consum/1  "Elec_power_W"
  Efficiency Map/1 -> MinMax/1
  MinMax1/1 -> Current_consum/2
  Constant/1 -> MinMax1/2
  Gain1/1 -> Saturation/1  "Mot_current_A"
  Switch/1 -> Switch1/1  "Elec_power_W"
  Constant1/1 -> Switch1/3

== system lib_EMachine/E-Machine/IMG Plant2/Thermal/Motor Thermal ==
  In1 : Inport
  Add1 : Sum  Inputs=+-
  Add2 : Sum
  Divide : Product  Inputs=*/
  Lower Limit : Subsystem  mask{Lolimit=t_amb+20}
      mask prompts: Lolimit "Lower Limit"
  Memory1 : Memory
  Motor Mass : Constant  Value=mot.plant.init.motor_mass
  Product : Product  RndMeth=Zero
  "Pump " : Constant  Value=0
  Specific Heat Cap Aluminum : Constant  Value=mot.plant.init.specific_heat
  tloop : Gain  Gain=tloop
  Out1 : Outport
  wires:
  Specific Heat Cap Aluminum/1 -> Product/2  "J/kg*K"
  Product/1 -> Divide/2
  Memory1/1 -> Add2/2
  Add2/1 -> Lower Limit/1(In1)
  Lower Limit/1(Out1) -> Out1/1, Memory1/1
  Divide/1 -> Add2/1
  tloop/1 -> Divide/1  "J"
  Motor Mass/1 -> Product/1  "kg"
  "Pump "/1 -> Add1/2
  In1/1 -> Add1/1
  Add1/1 -> tloop/1

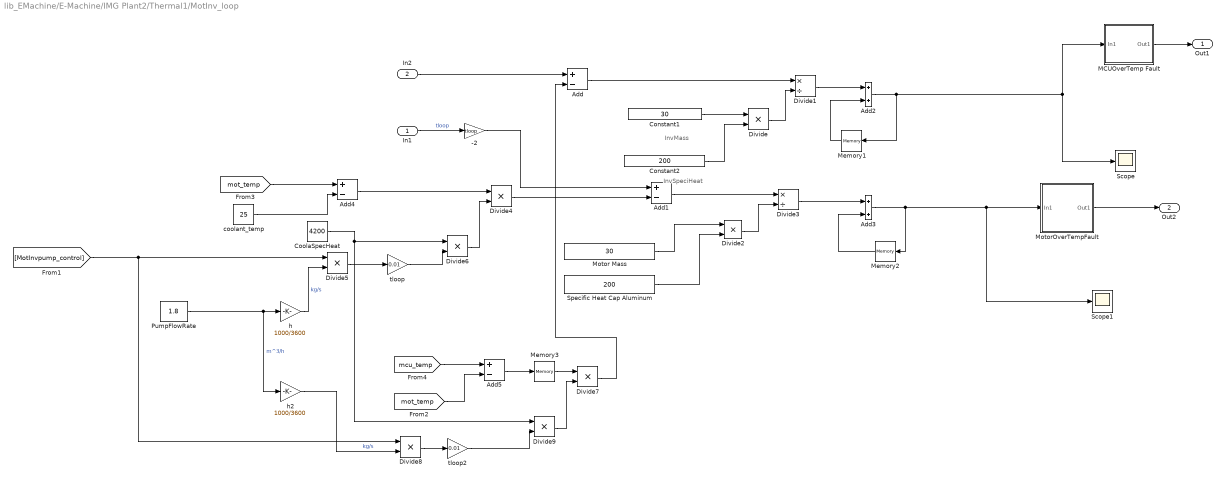
== system lib_EMachine/E-Machine/IMG Plant2/Thermal1/MotInv_loop ==
  note: InvSpeciHeat
  note: InvMass
  In1 : Inport
  In2 : Inport  Port=2
  -2 : Gain  Gain=tloop
  Add{,1,4..5} (4 alike) : Sum  Inputs=+-
  Add2 : Sum
  Add3 : Sum
  Constant1 : Constant  Value=30
  Constant2 : Constant  Value=200
  CoolaSpecHeat : Constant  Value=4200
  Divide{,2,4..9} (8 alike) : Product  Inputs=**
  Divide1 : Product  Inputs=*/
  Divide3 : Product  Inputs=*/
  MCUOverTemp Fault : Subsystem
  Memory1 : Memory  InitialCondition=25
  Memory2 : Memory  InitialCondition=25
  Memory3 : Memory
  Motor Mass : Constant  Value=30
  MotorOverTempFault : Subsystem
  PumpFlowRate : Constant  Value=1.8
  Scope : Scope
  Scope1 : Scope
  Specific Heat Cap Aluminum : Constant  Value=200
  coolant_temp : Constant  Value=25
  h : Gain  Gain=1000/3600
  h2 : Gain  Gain=1000/3600
  tloop : Gain  Gain=0.01
  tloop2 : Gain  Gain=0.01
  Out1 : Outport
  Out2 : Outport  Port=2
  wires:
  Add1/1 -> Divide3/1
  Memory1/1 -> Add2/2
  coolant_temp/1 -> Add4/2
  Divide/1 -> Divide1/2
  Specific Heat Cap Aluminum/1 -> Divide2/2
  Constant1/1 -> Divide/1
  Add/1 -> Divide1/1
  Memory2/1 -> Add3/2
  Add4/1 -> Divide4/1
  Add3/1 -> Scope1/1, MotorOverTempFault/1(In1), Memory2/1
  Divide6/1 -> Divide4/2
  Divide3/1 -> Add3/1
  Divide5/1 -> tloop/1
  Add2/1 -> MCUOverTemp Fault/1(In1), Scope/1, Memory1/1
  Divide2/1 -> Divide3/2
  Constant2/1 -> Divide/2
  Motor Mass/1 -> Divide2/1
  Divide1/1 -> Add2/1
  Divide7/1 -> Add/2
  h/1 -> Divide5/2  "kg/s"
  tloop/1 -> Divide6/2
  CoolaSpecHeat/1 -> Divide6/1, Divide9/1
  PumpFlowRate/1 -> h2/1, h/1  "m^3/h"
  h2/1 -> Divide8/2  "kg/s"
  Divide9/1 -> Divide7/2
  Divide8/1 -> tloop2/1
  tloop2/1 -> Divide9/2
  Divide4/1 -> Add1/2
  Add5/1 -> Memory3/1
  Memory3/1 -> Divide7/1
  MCUOverTemp Fault/1(Out1) -> Out1/1
  MotorOverTempFault/1(Out1) -> Out2/1
  [mot_temp] -> Add4/1
  [mcu_temp] -> Add5/1
  [mot_temp] -> Add5/2
  In1/1 -> -2/1  "tloop"
  In2/1 -> Add/1
  -2/1 -> Add1/1
  [MotInvpump_control] -> Divide8/1, Divide5/1

== system lib_EMachine/E-Machine/IMG Plant2/Thermal1/Motor Thermal ==
  In1 : Inport
  Add1 : Sum  Inputs=+-
  Add2 : Sum
  Divide : Product  Inputs=*/
  Lower Limit : Subsystem  mask{Lolimit=t_amb+20}
      mask prompts: Lolimit "Lower Limit"
  Memory1 : Memory
  Motor Mass : Constant  Value=mot.plant.init.motor_mass
  Product : Product  RndMeth=Zero
  "Pump " : Constant  Value=0
  Specific Heat Cap Aluminum : Constant  Value=mot.plant.init.specific_heat
  tloop : Gain  Gain=tloop
  Out1 : Outport
  wires:
  Specific Heat Cap Aluminum/1 -> Product/2  "J/kg*K"
  Product/1 -> Divide/2
  Memory1/1 -> Add2/2
  Add2/1 -> Lower Limit/1(In1)
  Lower Limit/1(Out1) -> Out1/1, Memory1/1
  Divide/1 -> Add2/1
  tloop/1 -> Divide/1  "J"
  Motor Mass/1 -> Product/1  "kg"
  "Pump "/1 -> Add1/2
  In1/1 -> Add1/1
  Add1/1 -> tloop/1

== system lib_EMachine/E-Machine/IMG Plant2/Torque Calculation/electric machine filter ==
  trq : Inport
  Interval Test : simulink/Logic and Bit Operations/Interval Test  IntervalClosedRight=on  uplimit=0.5  IntervalClosedLeft=on  lowlimit=-0.5  OutDataTypeStr=boolean
  Switch : Switch  Threshold=0.5
  electric machine time response : TransferFcn  Denominator=[mot.plant.init.time_response 1]
  filtered : Outport
  wires:
  electric machine time response/1 -> Switch/3
  Interval Test/1 -> Switch/2
  trq/1 -> Interval Test/1, electric machine time response/1, Switch/1
  Switch/1 -> filtered/1

== system lib_EMachine/E-Machine/IMG Plant2/Torque Calculation/max torque  ==
  cmd : Inport
  speed : Inport  Port=2
  Memory : Memory
  Peak trq max - Motoring : Lookup  InputValues=mot.plant.init.regen.trq_max.idx1_spd  Table=mot.plant.init.motor.trq_max.map  LookUpMeth=Interpolation-Use End Values  SaturateOnIntegerOverflow=on
  Peak trq max - Regen : Lookup  InputValues=mot.plant.init.regen.trq_max.idx1_spd  Table=mot.plant.init.regen.trq_max.map  LookUpMeth=Interpolation-Use End Values  SaturateOnIntegerOverflow=on
  Switch1 : Switch  SaturateOnIntegerOverflow=on
  rad/s  to RPM : Gain  Gain=30/pi
  max torque : Outport
  wires:
  Peak trq max - Motoring/1 -> Switch1/1
  speed/1 -> rad/s  to RPM/1
  cmd/1 -> Switch1/2
  Switch1/1 -> max torque/1
  Memory/1 -> Peak trq max - Motoring/1, Peak trq max - Regen/1
  rad/s  to RPM/1 -> Memory/1
  Peak trq max - Regen/1 -> Switch1/3

== system lib_EMachine/E-Machine/Soft MCU/Subsystem/MCU_RollingAliveCnt ==
  Counter Free-Running : simulink/Sources/Counter Free-Running  NumBits=4  tsamp=-1
  Out1 : Outport
  wires:
  Counter Free-Running/1 -> Out1/1  "MCURollingAliveCnt [0 1 2 3]"

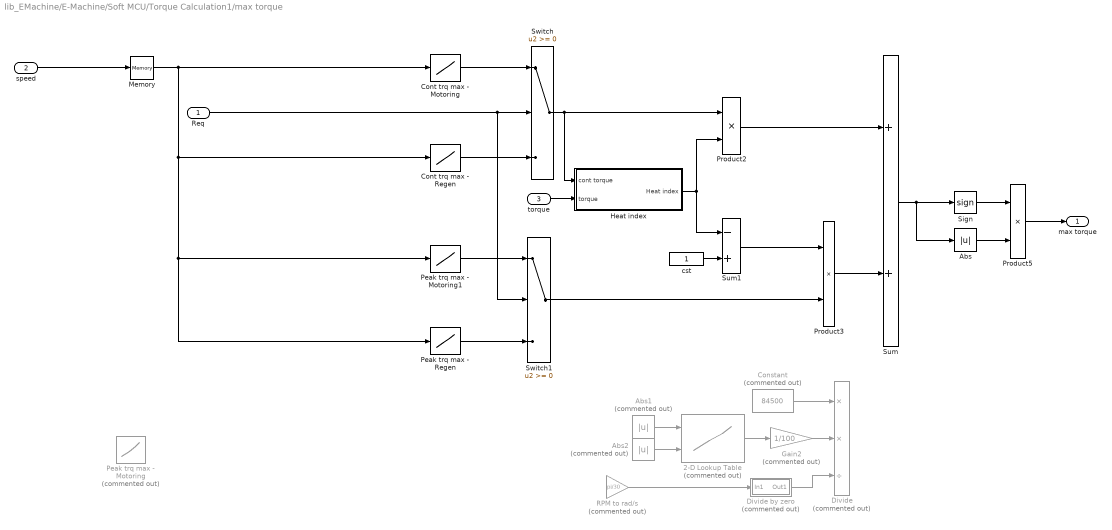
== system lib_EMachine/E-Machine/Soft MCU/Torque Calculation1/max torque  ==
  Req : Inport
  speed : Inport  Port=2
  torque : Inport  Port=3
  2-D Lookup Table : Lookup_n-D  Commented=on  BreakpointsForDimension1=mot.plant.init.eff_trq.idx2_trq  BreakpointsForDimension2=mot.plant.init.eff_trq.idx1_spd  Table=mot.plant.init.eff_trq.map  InternalRulePriority=Speed  RndMeth=Simplest  InputSameDT=on
  Abs : Abs  SaturateOnIntegerOverflow=on
  Abs1 : Abs  Commented=on
  Abs2 : Abs  Commented=on
  Constant : Constant  Commented=on  Value=84500
  Cont trq max - Motoring : Lookup  InputValues=mot.plant.init.motor.trq_cont.idx1_spd  Table=mot.plant.init.motor.trq_cont.map  LookUpMeth=Interpolation-Use End Values  SaturateOnIntegerOverflow=on
  Cont trq max - Regen : Lookup  InputValues=mot.plant.init.regen.trq_cont.idx1_spd  Table=mot.plant.init.regen.trq_cont.map  LookUpMeth=Interpolation-Use End Values  SaturateOnIntegerOverflow=on
  Divide : Product  Commented=on  Inputs=**/
  Divide by zero : Subsystem  Commented=on
  Gain2 : Gain  Commented=on  Gain=1/100
  Heat index : Subsystem
  Memory : Memory
  Peak trq max - Motoring : Lookup  Commented=on  InputValues=mot.plant.init.regen.trq_max.idx1_spd  Table=mot.plant.init.motor.trq_max.map  LookUpMeth=Interpolation-Use End Values  SaturateOnIntegerOverflow=on
  Peak trq max - Motoring1 : Lookup  InputValues=mot.plant.init.regen.trq_max.idx1_spd  Table=mot.plant.init.motor.trq_max.map  LookUpMeth=Interpolation-Use End Values  SaturateOnIntegerOverflow=on
  Peak trq max - Regen : Lookup  InputValues=mot.plant.init.regen.trq_max.idx1_spd  Table=mot.plant.init.regen.trq_max.map  LookUpMeth=Interpolation-Use End Values  SaturateOnIntegerOverflow=on
  Product2 : Product  SaturateOnIntegerOverflow=on  InputSameDT=on  OutDataTypeStr=Inherit: Same as first input
  Product3 : Product  SaturateOnIntegerOverflow=on  InputSameDT=on  OutDataTypeStr=Inherit: Same as first input
  Product5 : Product  SaturateOnIntegerOverflow=on  InputSameDT=on  OutDataTypeStr=Inherit: Same as first input
  RPM to rad/s : Gain  Commented=on  Gain=pi/30
  Sign : Signum
  Sum : Sum  SaturateOnIntegerOverflow=on  InputSameDT=on  OutDataTypeStr=Inherit: Same as first input
  Sum1 : Sum  Inputs=-+  SaturateOnIntegerOverflow=on  InputSameDT=on  OutDataTypeStr=Inherit: Same as first input
  Switch : Switch  SaturateOnIntegerOverflow=on
  Switch1 : Switch  SaturateOnIntegerOverflow=on
  cst : Constant
  max torque : Outport
  wires:
  Peak trq max - Motoring1/1 -> Switch1/1
  Divide by zero/1(Out1) -> Divide/3
  Req/1 -> Switch1/2, Switch/2
  Gain2/1 -> Divide/2
  2-D Lookup Table/1 -> Gain2/1
  Abs1/1 -> 2-D Lookup Table/1
  Abs2/1 -> 2-D Lookup Table/2
  RPM to rad/s/1 -> Divide by zero/1(In1)
  Constant/1 -> Divide/1
  speed/1 -> Memory/1
  Memory/1 -> Peak trq max - Regen/1, Peak trq max - Motoring1/1, Cont trq max - Regen/1, Cont trq max - Motoring/1
  Sign/1 -> Product5/1
  Product5/1 -> max torque/1
  Sum/1 -> Sign/1, Abs/1
  Abs/1 -> Product5/2
  torque/1 -> Heat index/2(torque)
  Cont trq max - Motoring/1 -> Switch/1
  Cont trq max - Regen/1 -> Switch/3
  Peak trq max - Regen/1 -> Switch1/3
  Switch/1 -> Product2/1, Heat index/1(cont torque)
  Switch1/1 -> Product3/2
  Product2/1 -> Sum/1
  Sum1/1 -> Product3/1
  Product3/1 -> Sum/2
  cst/1 -> Sum1/2
  Heat index/1(Heat index) -> Sum1/1, Product2/2

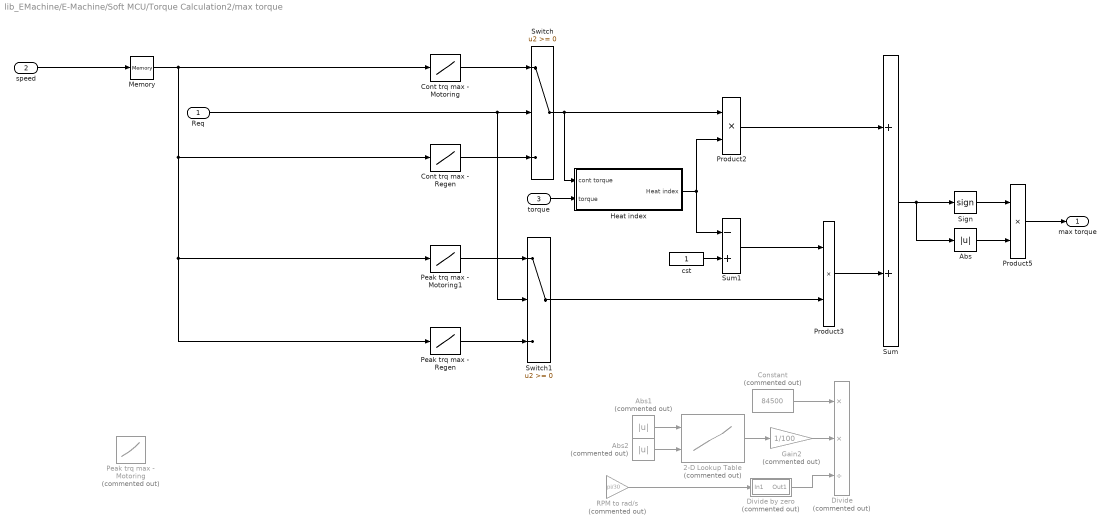
== system lib_EMachine/E-Machine/Soft MCU/Torque Calculation2/max torque  ==
  Req : Inport
  speed : Inport  Port=2
  torque : Inport  Port=3
  2-D Lookup Table : Lookup_n-D  Commented=on  BreakpointsForDimension1=mot.plant.init.eff_trq.idx2_trq  BreakpointsForDimension2=mot.plant.init.eff_trq.idx1_spd  Table=mot.plant.init.eff_trq.map  InternalRulePriority=Speed  RndMeth=Simplest  InputSameDT=on
  Abs : Abs  SaturateOnIntegerOverflow=on
  Abs1 : Abs  Commented=on
  Abs2 : Abs  Commented=on
  Constant : Constant  Commented=on  Value=84500
  Cont trq max - Motoring : Lookup  InputValues=mot.plant.init.motor.trq_cont.idx1_spd  Table=mot.plant.init.motor.trq_cont.map  LookUpMeth=Interpolation-Use End Values  SaturateOnIntegerOverflow=on
  Cont trq max - Regen : Lookup  InputValues=mot.plant.init.regen.trq_cont.idx1_spd  Table=mot.plant.init.regen.trq_cont.map  LookUpMeth=Interpolation-Use End Values  SaturateOnIntegerOverflow=on
  Divide : Product  Commented=on  Inputs=**/
  Divide by zero : Subsystem  Commented=on
  Gain2 : Gain  Commented=on  Gain=1/100
  Heat index : Subsystem
  Memory : Memory
  Peak trq max - Motoring : Lookup  Commented=on  InputValues=mot.plant.init.regen.trq_max.idx1_spd  Table=mot.plant.init.motor.trq_max.map  LookUpMeth=Interpolation-Use End Values  SaturateOnIntegerOverflow=on
  Peak trq max - Motoring1 : Lookup  InputValues=mot.plant.init.regen.trq_max.idx1_spd  Table=mot.plant.init.motor.trq_max.map  LookUpMeth=Interpolation-Use End Values  SaturateOnIntegerOverflow=on
  Peak trq max - Regen : Lookup  InputValues=mot.plant.init.regen.trq_max.idx1_spd  Table=mot.plant.init.regen.trq_max.map  LookUpMeth=Interpolation-Use End Values  SaturateOnIntegerOverflow=on
  Product2 : Product  SaturateOnIntegerOverflow=on  InputSameDT=on  OutDataTypeStr=Inherit: Same as first input
  Product3 : Product  SaturateOnIntegerOverflow=on  InputSameDT=on  OutDataTypeStr=Inherit: Same as first input
  Product5 : Product  SaturateOnIntegerOverflow=on  InputSameDT=on  OutDataTypeStr=Inherit: Same as first input
  RPM to rad/s : Gain  Commented=on  Gain=pi/30
  Sign : Signum
  Sum : Sum  SaturateOnIntegerOverflow=on  InputSameDT=on  OutDataTypeStr=Inherit: Same as first input
  Sum1 : Sum  Inputs=-+  SaturateOnIntegerOverflow=on  InputSameDT=on  OutDataTypeStr=Inherit: Same as first input
  Switch : Switch  SaturateOnIntegerOverflow=on
  Switch1 : Switch  SaturateOnIntegerOverflow=on
  cst : Constant
  max torque : Outport
  wires:
  Peak trq max - Motoring1/1 -> Switch1/1
  Divide by zero/1(Out1) -> Divide/3
  Req/1 -> Switch1/2, Switch/2
  Gain2/1 -> Divide/2
  2-D Lookup Table/1 -> Gain2/1
  Abs1/1 -> 2-D Lookup Table/1
  Abs2/1 -> 2-D Lookup Table/2
  RPM to rad/s/1 -> Divide by zero/1(In1)
  Constant/1 -> Divide/1
  speed/1 -> Memory/1
  Memory/1 -> Peak trq max - Regen/1, Peak trq max - Motoring1/1, Cont trq max - Regen/1, Cont trq max - Motoring/1
  Sign/1 -> Product5/1
  Product5/1 -> max torque/1
  Sum/1 -> Sign/1, Abs/1
  Abs/1 -> Product5/2
  torque/1 -> Heat index/2(torque)
  Cont trq max - Motoring/1 -> Switch/1
  Cont trq max - Regen/1 -> Switch/3
  Peak trq max - Regen/1 -> Switch1/3
  Switch/1 -> Product2/1, Heat index/1(cont torque)
  Switch1/1 -> Product3/2
  Product2/1 -> Sum/1
  Sum1/1 -> Product3/1
  Product3/1 -> Sum/2
  cst/1 -> Sum1/2
  Heat index/1(Heat index) -> Sum1/1, Product2/2

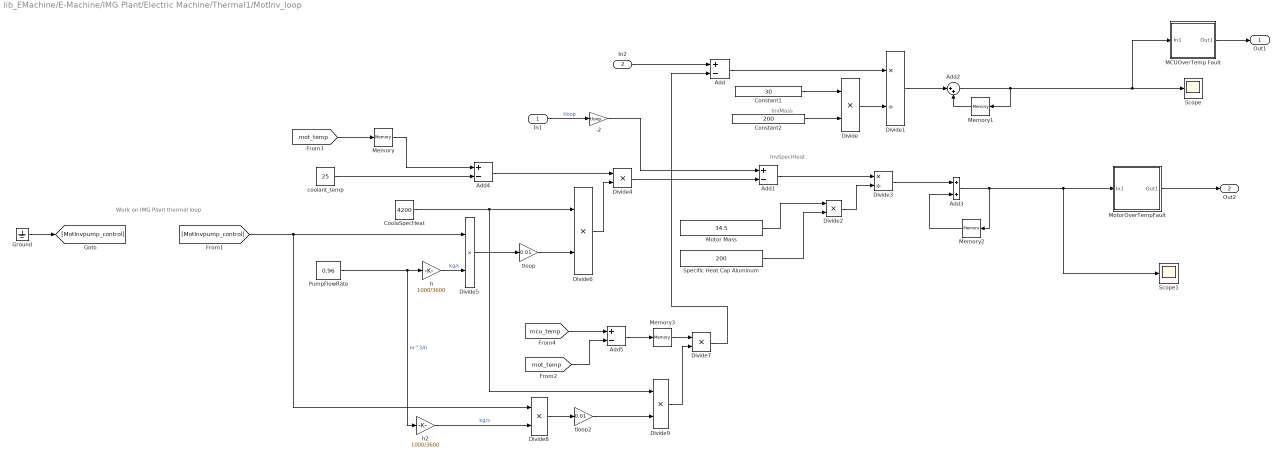
== system lib_EMachine/E-Machine/IMG Plant/Electric Machine/Thermal1/MotInv_loop ==
  note: InvSpeciHeat
  note: InvMass
  note: Work on IMG Plant thermal loop
  In1 : Inport
  In2 : Inport  Port=2
  -2 : Gain  Gain=tloop
  Add{,1,4..5} (4 alike) : Sum  Inputs=+-
  Add2 : Sum  Inputs=|++
  Add3 : Sum
  Constant1 : Constant  Value=30
  Constant2 : Constant  Value=200
  CoolaSpecHeat : Constant  Value=4200
  Divide{,2,4..9} (8 alike) : Product  Inputs=**
  Divide1 : Product  Inputs=*/
  Divide3 : Product  Inputs=*/
  Ground : Ground
  MCUOverTemp Fault : Subsystem
  Memory : Memory
  Memory1 : Memory  InitialCondition=25
  Memory2 : Memory  InitialCondition=25
  Memory3 : Memory
  Motor Mass : Constant  Value=34.5
  MotorOverTempFault : Subsystem
  PumpFlowRate : Constant  Value=0.96
  Scope : Scope
  Scope1 : Scope
  Specific Heat Cap Aluminum : Constant  Value=200
  coolant_temp : Constant  Value=25
  h : Gain  Gain=1000/3600
  h2 : Gain  Gain=1000/3600
  tloop : Gain  Gain=0.01
  tloop2 : Gain  Gain=0.01
  Out1 : Outport
  Out2 : Outport  Port=2
  wires:
  Ground/1 -> [MotInvpump_control]
  Memory/1 -> Add4/1
  Add1/1 -> Divide3/1
  Memory1/1 -> Add2/2
  coolant_temp/1 -> Add4/2
  Divide/1 -> Divide1/2
  Specific Heat Cap Aluminum/1 -> Divide2/2
  Constant1/1 -> Divide/1
  Add/1 -> Divide1/1
  Memory2/1 -> Add3/2
  Add4/1 -> Divide4/1
  Add3/1 -> Scope1/1, MotorOverTempFault/1(In1), Memory2/1
  Divide6/1 -> Divide4/2
  Divide3/1 -> Add3/1
  Divide5/1 -> tloop/1
  Add2/1 -> MCUOverTemp Fault/1(In1), Scope/1, Memory1/1
  Divide2/1 -> Divide3/2
  Constant2/1 -> Divide/2
  Motor Mass/1 -> Divide2/1
  Divide1/1 -> Add2/1
  Divide7/1 -> Add/2
  h/1 -> Divide5/2  "kg/s"
  tloop/1 -> Divide6/2
  CoolaSpecHeat/1 -> Divide6/1, Divide9/1
  PumpFlowRate/1 -> h/1, h2/1  "m^3/h"
  h2/1 -> Divide8/2  "kg/s"
  Divide9/1 -> Divide7/2
  Divide8/1 -> tloop2/1
  tloop2/1 -> Divide9/2
  Divide4/1 -> Add1/2
  Add5/1 -> Memory3/1
  Memory3/1 -> Divide7/1
  MCUOverTemp Fault/1(Out1) -> Out1/1
  MotorOverTempFault/1(Out1) -> Out2/1
  [mot_temp] -> Memory/1
  [mcu_temp] -> Add5/1
  [mot_temp] -> Add5/2
  In1/1 -> -2/1  "tloop"
  In2/1 -> Add/1
  -2/1 -> Add1/1
  [MotInvpump_control] -> Divide5/1, Divide8/1

== system lib_EMachine/E-Machine/IMG Plant/Electric Machine/Thermal1/Motor Thermal ==
  In1 : Inport
  Add1 : Sum  Inputs=+-
  Add2 : Sum
  Divide : Product  Inputs=*/
  Lower Limit : Subsystem  mask{Lolimit=t_amb+20}
      mask prompts: Lolimit "Lower Limit"
  Memory1 : Memory
  Motor Mass : Constant  Value=mot.plant.init.motor_mass
  Product : Product  RndMeth=Zero
  "Pump " : Constant  Value=0
  Specific Heat Cap Aluminum : Constant  Value=mot.plant.init.specific_heat
  tloop : Gain  Gain=tloop
  Out1 : Outport
  wires:
  Specific Heat Cap Aluminum/1 -> Product/2  "J/kg*K"
  Product/1 -> Divide/2
  Memory1/1 -> Add2/2
  Add2/1 -> Lower Limit/1(In1)
  Lower Limit/1(Out1) -> Out1/1, Memory1/1
  Divide/1 -> Add2/1
  tloop/1 -> Divide/1  "J"
  Motor Mass/1 -> Product/1  "kg"
  "Pump "/1 -> Add1/2
  In1/1 -> Add1/1
  Add1/1 -> tloop/1

== system lib_EMachine/E-Machine/IMG Plant/Electric Machine/Torque Calculation1/electric machine filter ==
  trq : Inport
  Interval Test : simulink/Logic and Bit Operations/Interval Test  IntervalClosedRight=on  uplimit=0.5  IntervalClosedLeft=on  lowlimit=-0.5  OutDataTypeStr=boolean
  Switch : Switch  Threshold=0.5
  electric machine time response : TransferFcn  Denominator=[mot.plant.init.time_response 1]
  filtered : Outport
  wires:
  electric machine time response/1 -> Switch/3
  Interval Test/1 -> Switch/2
  trq/1 -> Interval Test/1, electric machine time response/1, Switch/1
  Switch/1 -> filtered/1

== system lib_EMachine/E-Machine/IMG Plant/Electric Machine/Torque Calculation1/max torque  ==
  cmd : Inport
  speed : Inport  Port=2
  Memory : Memory
  Peak trq max - Motoring : Lookup  InputValues=mot.plant.init.regen.trq_max.idx1_spd  Table=mot.plant.init.motor.trq_max.map  LookUpMeth=Interpolation-Use End Values  SaturateOnIntegerOverflow=on
  Peak trq max - Regen : Lookup  InputValues=mot.plant.init.regen.trq_max.idx1_spd  Table=mot.plant.init.regen.trq_max.map  LookUpMeth=Interpolation-Use End Values  SaturateOnIntegerOverflow=on
  Switch1 : Switch  SaturateOnIntegerOverflow=on
  rad/s  to RPM : Gain  Gain=30/pi
  max torque : Outport
  wires:
  Peak trq max - Motoring/1 -> Switch1/1
  speed/1 -> rad/s  to RPM/1
  cmd/1 -> Switch1/2
  Switch1/1 -> max torque/1
  Memory/1 -> Peak trq max - Motoring/1, Peak trq max - Regen/1
  rad/s  to RPM/1 -> Memory/1
  Peak trq max - Regen/1 -> Switch1/3

== system lib_EMachine/E-Machine/IMG Plant2/Thermal/Motor Thermal/Lower Limit ==
  In1 : Inport
  Constant3 : Constant  Value=Lolimit
  MinMax : MinMax  Function=max  Inputs=2
  Out1 : Outport
  wires:
  In1/1 -> MinMax/1
  Constant3/1 -> MinMax/2
  MinMax/1 -> Out1/1

== system lib_EMachine/E-Machine/IMG Plant2/Thermal1/MotInv_loop/MCUOverTemp Fault ==
  In1 : Inport
  Gain : Gain  Gain=3
  Switch : Switch  Threshold=1
  Out1 : Outport
  wires:
  In1/1 -> Switch/3, Gain/1
  [MCUOverTemp] -> Switch/2
  Gain/1 -> Switch/1
  Switch/1 -> Out1/1

== system lib_EMachine/E-Machine/IMG Plant2/Thermal1/MotInv_loop/MotorOverTempFault ==
  In1 : Inport
  Gain : Gain  Gain=2
  Switch1 : Switch  Threshold=1
  Out1 : Outport
  wires:
  In1/1 -> Gain/1, Switch1/3
  [MotOverTemp] -> Switch1/2
  Gain/1 -> Switch1/1
  Switch1/1 -> Out1/1

== system lib_EMachine/E-Machine/IMG Plant2/Thermal1/Motor Thermal/Lower Limit ==
  In1 : Inport
  Constant3 : Constant  Value=Lolimit
  MinMax : MinMax  Function=max  Inputs=2
  Out1 : Outport
  wires:
  In1/1 -> MinMax/1
  Constant3/1 -> MinMax/2
  MinMax/1 -> Out1/1

== system lib_EMachine/E-Machine/Soft MCU/Torque Calculation1/max torque /Divide by zero ==
  In1 : Inport
  Compare To Constant : simulink/Logic and Bit Operations/Compare To Constant  relop===  const=0  OutDataTypeStr=boolean
  Constant1 : Constant
  Switch2 : Switch  Criteria=u2 > Threshold
  Out1 : Outport
  wires:
  Switch2/1 -> Out1/1
  In1/1 -> Compare To Constant/1, Switch2/3
  Compare To Constant/1 -> Switch2/2
  Constant1/1 -> Switch2/1
